simulink model "fuzzytesterunstable"  (R2018b)
settings: Solver=VariableStepAuto  StartTime=0.0  StopTime=10  RelTol=1e-3
libraries: fuzblock x2
settings Model: Creator=Nick  LastModifiedBy=Nick
settings SolverCC: ZeroCrossAlgorithm=Adaptive
settings DebuggingCC: IgnoredZcDiagnostic=none

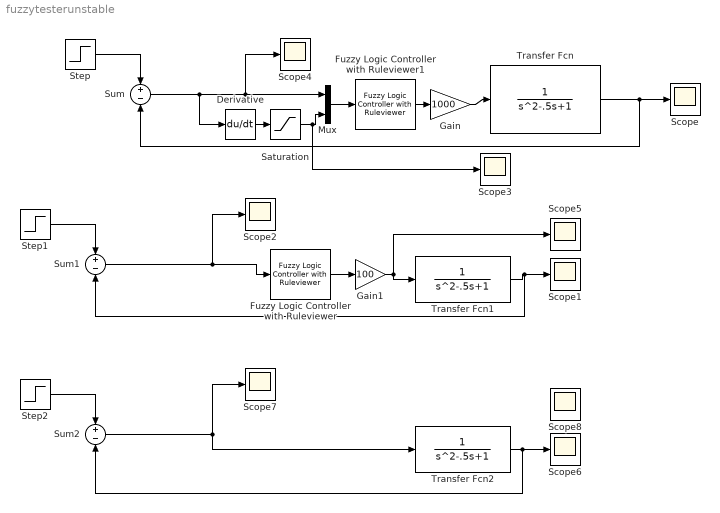
== system fuzzytesterunstable ==
  Derivative : Derivative
  Fuzzy Logic Controller with Ruleviewer : fuzblock/Fuzzy Logic  Controller  with Ruleviewer  fismatrix=fuzzyonlyerror  Ts=2
  Fuzzy Logic Controller with Ruleviewer1 : fuzblock/Fuzzy Logic  Controller  with Ruleviewer  fismatrix=fuzzyerder  Ts=2
  Gain : Gain  Gain=1000
  Gain1 : Gain  Gain=100
  Mux : Mux  Inputs=2
  Saturation : Saturate  UpperLimit=10  LowerLimit=-10
  Scope{,1..8} (9 alike) : Scope
  Step : Step  Time=0  SampleTime=0
  Step1 : Step  Time=0  SampleTime=0
  Step2 : Step  Time=0  SampleTime=0
  Sum : Sum  Inputs=+-
  Sum1 : Sum  Inputs=+-
  Sum2 : Sum  Inputs=+-
  Transfer Fcn : TransferFcn  Denominator=[1 -.5 1]
  Transfer Fcn1 : TransferFcn  Denominator=[1 -.5 1]
  Transfer Fcn2 : TransferFcn  Denominator=[1 -.5 1]
  wires:
  Transfer Fcn/1 -> Sum/2, Scope/1
  Sum/1 -> Derivative/1, Scope4/1, Mux/1
  Fuzzy Logic Controller with Ruleviewer1/1 -> Gain/1
  Transfer Fcn1/1 -> Scope1/1, Sum1/2
  Saturation/1 -> Scope3/1, Mux/2
  Derivative/1 -> Saturation/1
  Mux/1 -> Fuzzy Logic Controller with Ruleviewer1/1
  Gain/1 -> Transfer Fcn/1
  Fuzzy Logic Controller with Ruleviewer/1 -> Gain1/1
  Gain1/1 -> Scope5/1, Transfer Fcn1/1
  Sum2/1 -> Transfer Fcn2/1, Scope7/1
  Step2/1 -> Sum2/1
  Transfer Fcn2/1 -> Scope6/1, Sum2/2
  Sum1/1 -> Fuzzy Logic Controller with Ruleviewer/1, Scope2/1
  Step/1 -> Sum/1
  Step1/1 -> Sum1/1
